simulink model "CM745A_Sci30CfgAndUse"  (R2013b)
settings: Solver=ode45  StartTime=0.0  StopTime=10.0  RelTol=1e-3
libraries: simulink x12
(part 3 of 3)

== system CM745A_Sci30CfgAndUse/Sci30CfgAndUse/Sci30CfgAndUsePer2/Sci30Transmit/If Action Subsystem1/While Iterator Subsystem/CopyRight2 ==

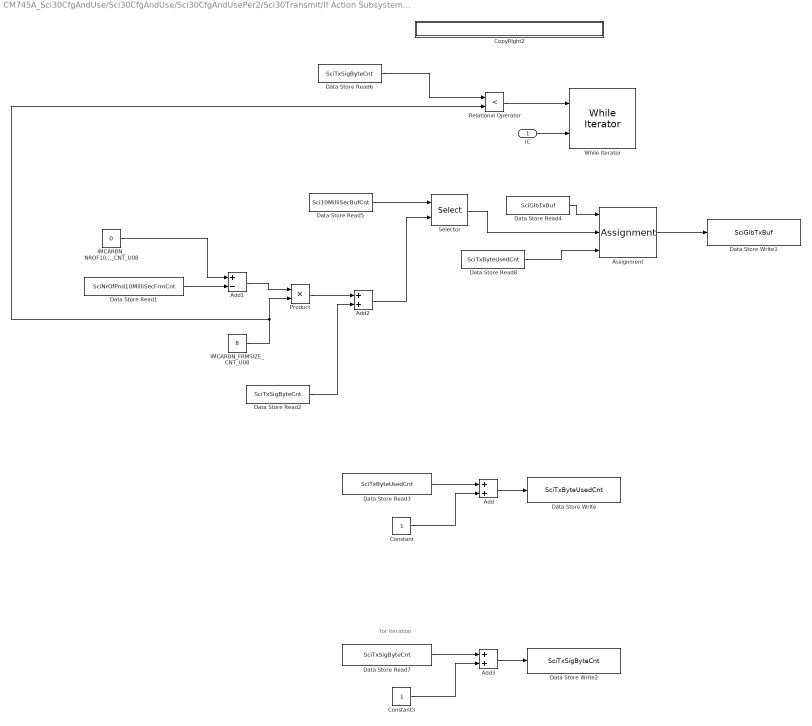
== system CM745A_Sci30CfgAndUse/Sci30CfgAndUse/Sci30CfgAndUsePer2/Sci30Transmit/If Action Subsystem1/While Iterator Subsystem/While Iterator Subsystem ==
  note: for iteration
  IC : Inport
  Add : Sum
  Add1 : Sum  Inputs=+-
  Add2 : Sum
  Add3 : Sum
  Assignment : Assignment  IndexMode=Zero-based  IndexOptions=Index vector (port)  Indices=1  OutputSizes=1
  Constant : Constant  OutDataTypeStr=uint8
  Constant3 : Constant  OutDataTypeStr=uint8
  CopyRight2 : Subsystem  Description=|  mask(Copyright Information){none=on}
      | Copyright info block.                                               
      |                                                                     
      | Place copyright information at the top of every subsystem in design.
      mask prompts: none "No parameters"
      mask help: Place copyright information at the top of every subsystem in design.
      mask Display:
      | NxtrConf = 'Nexteer Confidential';
      | 
      | sys = bdroot; %handle for the current model ("system")
      | first = get_param(sys,'Created');
      | first = first(end-3:end);  %year is last four digits
      | 
      | last = get_param(sys,'LastModifiedDate');
      | if isempty(last)
      |     last = datestr(now,'yyyy');
      | else
      |     last = last(end-3:end);
      | end
      | 
      | if strcmp(first,last)
      |     fprintf('%s -- Copyright %s Nexteer',NxtrConf,first)
      | else
      |     fprintf('%s -- %s%s- %s Nexteer',NxtrConf,char(169),first,last)
      | end
  Data Store Read1 : DataStoreRead  DataStoreName=SciNrOfPnd10MilliSecFrmCnt
  Data Store Read2 : DataStoreRead  DataStoreName=SciTxSigByteCnt
  Data Store Read3 : DataStoreRead  DataStoreName=SciTxByteUsedCnt
  Data Store Read4 : DataStoreRead  DataStoreName=SciGlbTxBuf
  Data Store Read5 : DataStoreRead  DataStoreName=Sci10MilliSecBufCnt
  Data Store Read6 : DataStoreRead  DataStoreName=SciTxSigByteCnt
  Data Store Read7 : DataStoreRead  DataStoreName=SciTxSigByteCnt
  Data Store Read8 : DataStoreRead  DataStoreName=SciTxByteUsedCnt
  Data Store Write : DataStoreWrite  DataStoreName=SciTxByteUsedCnt
  Data Store Write1 : DataStoreWrite  DataStoreName=SciGlbTxBuf
  Data Store Write2 : DataStoreWrite  DataStoreName=SciTxSigByteCnt
  IMCARBN_FRMSIZE_CNT_U08 : Constant  Value=8  OutDataTypeStr=uint8
  IMCARBN_NROF10MILLISECRATEGROUP_CNT_U08 : Constant  Value=0
  Product : Product
  Relational Operator : RelationalOperator  Operator=<  OutDataTypeStr=boolean
  Selector : Selector  IndexMode=Zero-based  InputPortWidth=2047  IndexOptions=Index vector (port)  Indices=[1 3]  OutputSizes=1
  While Iterator : WhileIterator  MaxIters=-1  ResetStates=reset
  wires:
  Data Store Read3/1 -> Add/1
  Add/1 -> Data Store Write/1
  Constant/1 -> Add/2
  Assignment/1 -> Data Store Write1/1
  Data Store Read4/1 -> Assignment/1
  Selector/1 -> Assignment/2
  Data Store Read5/1 -> Selector/1
  Add2/1 -> Selector/2
  IMCARBN_NROF10MILLISECRATEGROUP_CNT_U08/1 -> Add1/1
  Data Store Read1/1 -> Add1/2
  Add1/1 -> Product/1
  IMCARBN_FRMSIZE_CNT_U08/1 -> Relational Operator/2, Product/2
  Product/1 -> Add2/1
  Data Store Read2/1 -> Add2/2
  IC/1 -> While Iterator/2
  Data Store Read6/1 -> Relational Operator/1
  Relational Operator/1 -> While Iterator/1
  Data Store Read7/1 -> Add3/1
  Add3/1 -> Data Store Write2/1
  Constant3/1 -> Add3/2
  Data Store Read8/1 -> Assignment/3

== system CM745A_Sci30CfgAndUse/Sci30CfgAndUse/Sci30CfgAndUsePer2/Sci30Transmit/If Action Subsystem2/If Action Subsystem/CopyRight2 ==

== system CM745A_Sci30CfgAndUse/Sci30CfgAndUse/Sci30CfgAndUsePer2/Sci30Transmit/If Action Subsystem2/While Iterator Subsystem/CopyRight2 ==

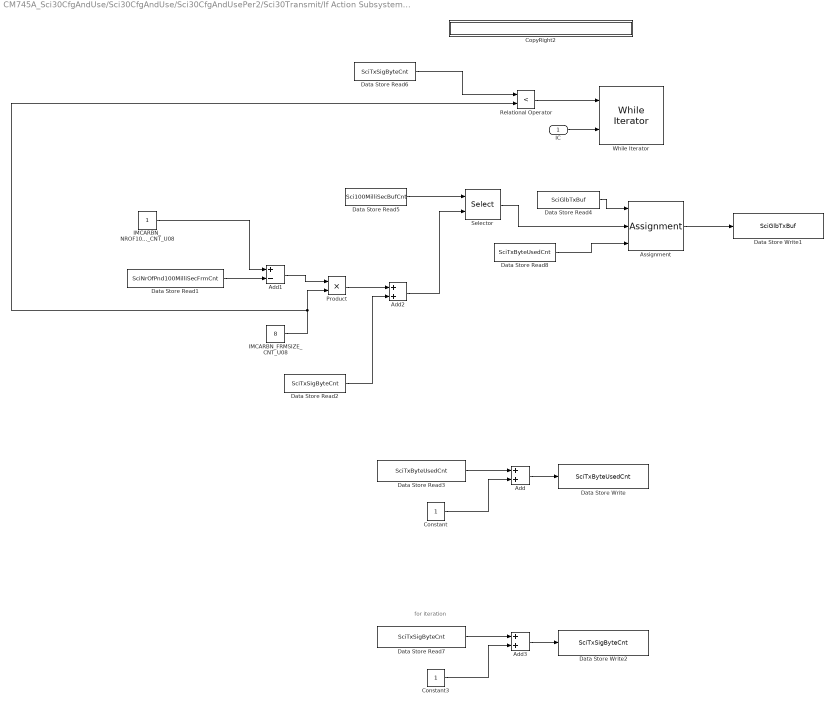
== system CM745A_Sci30CfgAndUse/Sci30CfgAndUse/Sci30CfgAndUsePer2/Sci30Transmit/If Action Subsystem2/While Iterator Subsystem/While Iterator Subsystem ==
  note: for iteration
  IC : Inport
  Add : Sum
  Add1 : Sum  Inputs=+-
  Add2 : Sum
  Add3 : Sum
  Assignment : Assignment  IndexMode=Zero-based  IndexOptions=Index vector (port)  Indices=1  OutputSizes=1
  Constant : Constant  OutDataTypeStr=uint8
  Constant3 : Constant  OutDataTypeStr=uint8
  CopyRight2 : Subsystem  Description=|  mask(Copyright Information){none=on}
      | Copyright info block.                                               
      |                                                                     
      | Place copyright information at the top of every subsystem in design.
      mask prompts: none "No parameters"
      mask help: Place copyright information at the top of every subsystem in design.
      mask Display:
      | NxtrConf = 'Nexteer Confidential';
      | 
      | sys = bdroot; %handle for the current model ("system")
      | first = get_param(sys,'Created');
      | first = first(end-3:end);  %year is last four digits
      | 
      | last = get_param(sys,'LastModifiedDate');
      | if isempty(last)
      |     last = datestr(now,'yyyy');
      | else
      |     last = last(end-3:end);
      | end
      | 
      | if strcmp(first,last)
      |     fprintf('%s -- Copyright %s Nexteer',NxtrConf,first)
      | else
      |     fprintf('%s -- %s%s- %s Nexteer',NxtrConf,char(169),first,last)
      | end
  Data Store Read1 : DataStoreRead  DataStoreName=SciNrOfPnd100MilliSecFrmCnt
  Data Store Read2 : DataStoreRead  DataStoreName=SciTxSigByteCnt
  Data Store Read3 : DataStoreRead  DataStoreName=SciTxByteUsedCnt
  Data Store Read4 : DataStoreRead  DataStoreName=SciGlbTxBuf
  Data Store Read5 : DataStoreRead  DataStoreName=Sci100MilliSecBufCnt
  Data Store Read6 : DataStoreRead  DataStoreName=SciTxSigByteCnt
  Data Store Read7 : DataStoreRead  DataStoreName=SciTxSigByteCnt
  Data Store Read8 : DataStoreRead  DataStoreName=SciTxByteUsedCnt
  Data Store Write : DataStoreWrite  DataStoreName=SciTxByteUsedCnt
  Data Store Write1 : DataStoreWrite  DataStoreName=SciGlbTxBuf
  Data Store Write2 : DataStoreWrite  DataStoreName=SciTxSigByteCnt
  IMCARBN_FRMSIZE_CNT_U08 : Constant  Value=8  OutDataTypeStr=uint8
  IMCARBN_NROF100MILLISECRATEGROUP_CNT_U08 : Constant
  Product : Product
  Relational Operator : RelationalOperator  Operator=<  OutDataTypeStr=boolean
  Selector : Selector  IndexMode=Zero-based  InputPortWidth=2047  IndexOptions=Index vector (port)  Indices=[1 3]  OutputSizes=1
  While Iterator : WhileIterator  MaxIters=-1  ResetStates=reset
  wires:
  Data Store Read3/1 -> Add/1
  Add/1 -> Data Store Write/1
  Constant/1 -> Add/2
  Assignment/1 -> Data Store Write1/1
  Data Store Read4/1 -> Assignment/1
  Selector/1 -> Assignment/2
  Data Store Read5/1 -> Selector/1
  Add2/1 -> Selector/2
  IMCARBN_NROF100MILLISECRATEGROUP_CNT_U08/1 -> Add1/1
  Data Store Read1/1 -> Add1/2
  Add1/1 -> Product/1
  IMCARBN_FRMSIZE_CNT_U08/1 -> Relational Operator/2, Product/2
  Product/1 -> Add2/1
  Data Store Read2/1 -> Add2/2
  IC/1 -> While Iterator/2
  Data Store Read6/1 -> Relational Operator/1
  Relational Operator/1 -> While Iterator/1
  Data Store Read7/1 -> Add3/1
  Add3/1 -> Data Store Write2/1
  Constant3/1 -> Add3/2
  Data Store Read8/1 -> Assignment/3

== system CM745A_Sci30CfgAndUse/Sci30CfgAndUse/Sci30CfgAndUsePer2/Sci30Transmit/Update DTS registers/If Action Subsystem/CopyRight2 ==

== system CM745A_Sci30CfgAndUse/Sci30CfgAndUse/Sci30CfgAndUsePer1/If Action Subsystem2/While Iterator Subsystem/If Action Subsystem/If Action Subsystem/CopyRight2 ==

== system CM745A_Sci30CfgAndUse/Sci30CfgAndUse/Sci30CfgAndUsePer1/If Action Subsystem2/While Iterator Subsystem/If Action Subsystem/If Action Subsystem1/CopyRight2 ==

== system CM745A_Sci30CfgAndUse/Sci30CfgAndUse/Sci30CfgAndUsePer1/If Action Subsystem2/While Iterator Subsystem/If Action Subsystem/If Action Subsystem1/RollovrAdd ==
  In1 : Inport
  In2 : Inport  Port=2
  Add : Sum
  Constant : Constant  Value=2  OutDataTypeStr=uint8
  CopyRight2 : Subsystem  Description=|  mask(Copyright Information){none=on}
      | Copyright info block.                                               
      |                                                                     
      | Place copyright information at the top of every subsystem in design.
      mask prompts: none "No parameters"
      mask help: Place copyright information at the top of every subsystem in design.
      mask Display:
      | NxtrConf = 'Nexteer Confidential';
      | 
      | sys = bdroot; %handle for the current model ("system")
      | first = get_param(sys,'Created');
      | first = first(end-3:end);  %year is last four digits
      | 
      | last = get_param(sys,'LastModifiedDate');
      | if isempty(last)
      |     last = datestr(now,'yyyy');
      | else
      |     last = last(end-3:end);
      | end
      | 
      | if strcmp(first,last)
      |     fprintf('%s -- Copyright %s Nexteer',NxtrConf,first)
      | else
      |     fprintf('%s -- %s%s- %s Nexteer',NxtrConf,char(169),first,last)
      | end
  IMCARBN_FRMSIZE_CNT_U08 : Constant  Value=8  OutDataTypeStr=uint8
  MAXSIGGROUPFORTX_CNT_U08 : Constant  Value=9  OutDataTypeStr=uint8
  Math Function : Math  Operator=mod  SaturateOnIntegerOverflow=on
  Product : Product
  Product1 : Product  OutDataTypeStr=uint8
  Out1 : Outport
  wires:
  Math Function/1 -> Out1/1
  In1/1 -> Add/1
  In2/1 -> Add/2
  Add/1 -> Math Function/1
  Constant/1 -> Product/1
  IMCARBN_FRMSIZE_CNT_U08/1 -> Product/2
  Product/1 -> Product1/1
  Product1/1 -> Math Function/2
  MAXSIGGROUPFORTX_CNT_U08/1 -> Product1/2

== system CM745A_Sci30CfgAndUse/Sci30CfgAndUse/Sci30CfgAndUsePer1/If Action Subsystem2/While Iterator Subsystem/If Action Subsystem/If Action Subsystem2/CopyRight2 ==

== system CM745A_Sci30CfgAndUse/Sci30CfgAndUse/Sci30CfgAndUsePer1/If Action Subsystem2/While Iterator Subsystem/If Action Subsystem/If Action Subsystem2/RollovrAdd ==
  In1 : Inport
  In2 : Inport  Port=2
  Add : Sum
  Constant : Constant  Value=2  OutDataTypeStr=uint8
  CopyRight2 : Subsystem  Description=|  mask(Copyright Information){none=on}
      | Copyright info block.                                               
      |                                                                     
      | Place copyright information at the top of every subsystem in design.
      mask prompts: none "No parameters"
      mask help: Place copyright information at the top of every subsystem in design.
      mask Display:
      | NxtrConf = 'Nexteer Confidential';
      | 
      | sys = bdroot; %handle for the current model ("system")
      | first = get_param(sys,'Created');
      | first = first(end-3:end);  %year is last four digits
      | 
      | last = get_param(sys,'LastModifiedDate');
      | if isempty(last)
      |     last = datestr(now,'yyyy');
      | else
      |     last = last(end-3:end);
      | end
      | 
      | if strcmp(first,last)
      |     fprintf('%s -- Copyright %s Nexteer',NxtrConf,first)
      | else
      |     fprintf('%s -- %s%s- %s Nexteer',NxtrConf,char(169),first,last)
      | end
  IMCARBN_FRMSIZE_CNT_U08 : Constant  Value=8
  MAXSIGGROUPFORTX_CNT_U08 : Constant  Value=9
  Math Function : Math  Operator=mod  SaturateOnIntegerOverflow=on
  Product : Product  OutDataTypeStr=uint8
  Product1 : Product  OutDataTypeStr=uint8
  Out1 : Outport
  wires:
  Math Function/1 -> Out1/1
  In1/1 -> Add/1
  In2/1 -> Add/2
  Add/1 -> Math Function/1
  Constant/1 -> Product/1
  IMCARBN_FRMSIZE_CNT_U08/1 -> Product/2
  Product/1 -> Product1/1
  Product1/1 -> Math Function/2
  MAXSIGGROUPFORTX_CNT_U08/1 -> Product1/2

== system CM745A_Sci30CfgAndUse/Sci30CfgAndUse/Sci30CfgAndUsePer1/If Action Subsystem2/While Iterator Subsystem/If Action Subsystem/If Action Subsystem2/RollovrAdd1 ==
  In1 : Inport
  In2 : Inport  Port=2
  Add : Sum
  Constant : Constant  Value=2  OutDataTypeStr=uint8
  CopyRight2 : Subsystem  Description=|  mask(Copyright Information){none=on}
      | Copyright info block.                                               
      |                                                                     
      | Place copyright information at the top of every subsystem in design.
      mask prompts: none "No parameters"
      mask help: Place copyright information at the top of every subsystem in design.
      mask Display:
      | NxtrConf = 'Nexteer Confidential';
      | 
      | sys = bdroot; %handle for the current model ("system")
      | first = get_param(sys,'Created');
      | first = first(end-3:end);  %year is last four digits
      | 
      | last = get_param(sys,'LastModifiedDate');
      | if isempty(last)
      |     last = datestr(now,'yyyy');
      | else
      |     last = last(end-3:end);
      | end
      | 
      | if strcmp(first,last)
      |     fprintf('%s -- Copyright %s Nexteer',NxtrConf,first)
      | else
      |     fprintf('%s -- %s%s- %s Nexteer',NxtrConf,char(169),first,last)
      | end
  IMCARBN_FRMSIZE_CNT_U08 : Constant  Value=8
  MAXSIGGROUPFORTX_CNT_U08 : Constant  Value=9
  Math Function : Math  Operator=mod  SaturateOnIntegerOverflow=on
  Product : Product
  Product1 : Product
  Out1 : Outport
  wires:
  Math Function/1 -> Out1/1
  In1/1 -> Add/1
  In2/1 -> Add/2
  Add/1 -> Math Function/1
  Constant/1 -> Product/1
  IMCARBN_FRMSIZE_CNT_U08/1 -> Product/2
  Product/1 -> Product1/1
  Product1/1 -> Math Function/2
  MAXSIGGROUPFORTX_CNT_U08/1 -> Product1/2

== system CM745A_Sci30CfgAndUse/Sci30CfgAndUse/Sci30CfgAndUsePer1/If Action Subsystem2/While Iterator Subsystem/If Action Subsystem/If Action Subsystem2/RollovrAdd2 ==
  In1 : Inport
  In2 : Inport  Port=2
  Add : Sum
  Constant : Constant  Value=2  OutDataTypeStr=uint8
  CopyRight2 : Subsystem  Description=|  mask(Copyright Information){none=on}
      | Copyright info block.                                               
      |                                                                     
      | Place copyright information at the top of every subsystem in design.
      mask prompts: none "No parameters"
      mask help: Place copyright information at the top of every subsystem in design.
      mask Display:
      | NxtrConf = 'Nexteer Confidential';
      | 
      | sys = bdroot; %handle for the current model ("system")
      | first = get_param(sys,'Created');
      | first = first(end-3:end);  %year is last four digits
      | 
      | last = get_param(sys,'LastModifiedDate');
      | if isempty(last)
      |     last = datestr(now,'yyyy');
      | else
      |     last = last(end-3:end);
      | end
      | 
      | if strcmp(first,last)
      |     fprintf('%s -- Copyright %s Nexteer',NxtrConf,first)
      | else
      |     fprintf('%s -- %s%s- %s Nexteer',NxtrConf,char(169),first,last)
      | end
  IMCARBN_FRMSIZE_CNT_U08 : Constant  Value=8
  MAXSIGGROUPFORTX_CNT_U08 : Constant  Value=9
  Math Function : Math  Operator=mod  SaturateOnIntegerOverflow=on
  Product : Product
  Product1 : Product
  Out1 : Outport
  wires:
  MAXSIGGROUPFORTX_CNT_U08/1 -> Product1/2
  Product1/1 -> Math Function/2
  Product/1 -> Product1/1
  IMCARBN_FRMSIZE_CNT_U08/1 -> Product/2
  Constant/1 -> Product/1
  Add/1 -> Math Function/1
  In2/1 -> Add/2
  In1/1 -> Add/1
  Math Function/1 -> Out1/1

== system CM745A_Sci30CfgAndUse/Sci30CfgAndUse/Sci30CfgAndUsePer1/If Action Subsystem2/While Iterator Subsystem/If Action Subsystem/If Action Subsystem2/RollovrAdd3 ==
  In1 : Inport
  In2 : Inport  Port=2
  Add : Sum
  Constant : Constant  Value=2  OutDataTypeStr=uint8
  CopyRight2 : Subsystem  Description=|  mask(Copyright Information){none=on}
      | Copyright info block.                                               
      |                                                                     
      | Place copyright information at the top of every subsystem in design.
      mask prompts: none "No parameters"
      mask help: Place copyright information at the top of every subsystem in design.
      mask Display:
      | NxtrConf = 'Nexteer Confidential';
      | 
      | sys = bdroot; %handle for the current model ("system")
      | first = get_param(sys,'Created');
      | first = first(end-3:end);  %year is last four digits
      | 
      | last = get_param(sys,'LastModifiedDate');
      | if isempty(last)
      |     last = datestr(now,'yyyy');
      | else
      |     last = last(end-3:end);
      | end
      | 
      | if strcmp(first,last)
      |     fprintf('%s -- Copyright %s Nexteer',NxtrConf,first)
      | else
      |     fprintf('%s -- %s%s- %s Nexteer',NxtrConf,char(169),first,last)
      | end
  IMCARBN_FRMSIZE_CNT_U08 : Constant  Value=8
  MAXSIGGROUPFORTX_CNT_U08 : Constant  Value=9
  Math Function : Math  Operator=mod  SaturateOnIntegerOverflow=on
  Product : Product
  Product1 : Product
  Out1 : Outport
  wires:
  Math Function/1 -> Out1/1
  In1/1 -> Add/1
  In2/1 -> Add/2
  Add/1 -> Math Function/1
  Constant/1 -> Product/1
  IMCARBN_FRMSIZE_CNT_U08/1 -> Product/2
  Product/1 -> Product1/1
  Product1/1 -> Math Function/2
  MAXSIGGROUPFORTX_CNT_U08/1 -> Product1/2

== system CM745A_Sci30CfgAndUse/Sci30CfgAndUse/Sci30CfgAndUsePer1/If Action Subsystem2/While Iterator Subsystem/If Action Subsystem/If Action Subsystem2/RollovrAdd4 ==
  In1 : Inport
  In2 : Inport  Port=2
  Add : Sum
  Constant : Constant  Value=2  OutDataTypeStr=uint8
  CopyRight2 : Subsystem  Description=|  mask(Copyright Information){none=on}
      | Copyright info block.                                               
      |                                                                     
      | Place copyright information at the top of every subsystem in design.
      mask prompts: none "No parameters"
      mask help: Place copyright information at the top of every subsystem in design.
      mask Display:
      | NxtrConf = 'Nexteer Confidential';
      | 
      | sys = bdroot; %handle for the current model ("system")
      | first = get_param(sys,'Created');
      | first = first(end-3:end);  %year is last four digits
      | 
      | last = get_param(sys,'LastModifiedDate');
      | if isempty(last)
      |     last = datestr(now,'yyyy');
      | else
      |     last = last(end-3:end);
      | end
      | 
      | if strcmp(first,last)
      |     fprintf('%s -- Copyright %s Nexteer',NxtrConf,first)
      | else
      |     fprintf('%s -- %s%s- %s Nexteer',NxtrConf,char(169),first,last)
      | end
  IMCARBN_FRMSIZE_CNT_U08 : Constant  Value=8
  MAXSIGGROUPFORTX_CNT_U08 : Constant  Value=9
  Math Function : Math  Operator=mod  SaturateOnIntegerOverflow=on
  Product : Product
  Product1 : Product
  Out1 : Outport
  wires:
  MAXSIGGROUPFORTX_CNT_U08/1 -> Product1/2
  Product1/1 -> Math Function/2
  Product/1 -> Product1/1
  IMCARBN_FRMSIZE_CNT_U08/1 -> Product/2
  Constant/1 -> Product/1
  Add/1 -> Math Function/1
  In2/1 -> Add/2
  In1/1 -> Add/1
  Math Function/1 -> Out1/1

== system CM745A_Sci30CfgAndUse/Sci30CfgAndUse/Sci30CfgAndUsePer1/If Action Subsystem2/While Iterator Subsystem/If Action Subsystem/If Action Subsystem2/RollovrAdd5 ==
  In1 : Inport
  In2 : Inport  Port=2
  Add : Sum
  Constant : Constant  Value=2  OutDataTypeStr=uint8
  CopyRight2 : Subsystem  Description=|  mask(Copyright Information){none=on}
      | Copyright info block.                                               
      |                                                                     
      | Place copyright information at the top of every subsystem in design.
      mask prompts: none "No parameters"
      mask help: Place copyright information at the top of every subsystem in design.
      mask Display:
      | NxtrConf = 'Nexteer Confidential';
      | 
      | sys = bdroot; %handle for the current model ("system")
      | first = get_param(sys,'Created');
      | first = first(end-3:end);  %year is last four digits
      | 
      | last = get_param(sys,'LastModifiedDate');
      | if isempty(last)
      |     last = datestr(now,'yyyy');
      | else
      |     last = last(end-3:end);
      | end
      | 
      | if strcmp(first,last)
      |     fprintf('%s -- Copyright %s Nexteer',NxtrConf,first)
      | else
      |     fprintf('%s -- %s%s- %s Nexteer',NxtrConf,char(169),first,last)
      | end
  IMCARBN_FRMSIZE_CNT_U08 : Constant  Value=8
  MAXSIGGROUPFORTX_CNT_U08 : Constant  Value=9
  Math Function : Math  Operator=mod  SaturateOnIntegerOverflow=on
  Product : Product
  Product1 : Product
  Out1 : Outport
  wires:
  Math Function/1 -> Out1/1
  In1/1 -> Add/1
  In2/1 -> Add/2
  Add/1 -> Math Function/1
  Constant/1 -> Product/1
  IMCARBN_FRMSIZE_CNT_U08/1 -> Product/2
  Product/1 -> Product1/1
  Product1/1 -> Math Function/2
  MAXSIGGROUPFORTX_CNT_U08/1 -> Product1/2

== system CM745A_Sci30CfgAndUse/Sci30CfgAndUse/Sci30CfgAndUsePer1/If Action Subsystem2/While Iterator Subsystem/If Action Subsystem/If Action Subsystem2/RollovrAdd6 ==
  In1 : Inport
  In2 : Inport  Port=2
  Add : Sum
  Constant : Constant  Value=2  OutDataTypeStr=uint8
  CopyRight2 : Subsystem  Description=|  mask(Copyright Information){none=on}
      | Copyright info block.                                               
      |                                                                     
      | Place copyright information at the top of every subsystem in design.
      mask prompts: none "No parameters"
      mask help: Place copyright information at the top of every subsystem in design.
      mask Display:
      | NxtrConf = 'Nexteer Confidential';
      | 
      | sys = bdroot; %handle for the current model ("system")
      | first = get_param(sys,'Created');
      | first = first(end-3:end);  %year is last four digits
      | 
      | last = get_param(sys,'LastModifiedDate');
      | if isempty(last)
      |     last = datestr(now,'yyyy');
      | else
      |     last = last(end-3:end);
      | end
      | 
      | if strcmp(first,last)
      |     fprintf('%s -- Copyright %s Nexteer',NxtrConf,first)
      | else
      |     fprintf('%s -- %s%s- %s Nexteer',NxtrConf,char(169),first,last)
      | end
  IMCARBN_FRMSIZE_CNT_U08 : Constant  Value=8
  MAXSIGGROUPFORTX_CNT_U08 : Constant  Value=9
  Math Function : Math  Operator=mod  SaturateOnIntegerOverflow=on
  Product : Product
  Product1 : Product
  Out1 : Outport
  wires:
  MAXSIGGROUPFORTX_CNT_U08/1 -> Product1/2
  Product1/1 -> Math Function/2
  Product/1 -> Product1/1
  IMCARBN_FRMSIZE_CNT_U08/1 -> Product/2
  Constant/1 -> Product/1
  Add/1 -> Math Function/1
  In2/1 -> Add/2
  In1/1 -> Add/1
  Math Function/1 -> Out1/1

== system CM745A_Sci30CfgAndUse/Sci30CfgAndUse/Sci30CfgAndUsePer1/If Action Subsystem2/While Iterator Subsystem/If Action Subsystem/If Action Subsystem2/RollovrAdd7 ==
  In1 : Inport
  In2 : Inport  Port=2
  Add : Sum
  Constant : Constant  Value=2  OutDataTypeStr=uint8
  CopyRight2 : Subsystem  Description=|  mask(Copyright Information){none=on}
      | Copyright info block.                                               
      |                                                                     
      | Place copyright information at the top of every subsystem in design.
      mask prompts: none "No parameters"
      mask help: Place copyright information at the top of every subsystem in design.
      mask Display:
      | NxtrConf = 'Nexteer Confidential';
      | 
      | sys = bdroot; %handle for the current model ("system")
      | first = get_param(sys,'Created');
      | first = first(end-3:end);  %year is last four digits
      | 
      | last = get_param(sys,'LastModifiedDate');
      | if isempty(last)
      |     last = datestr(now,'yyyy');
      | else
      |     last = last(end-3:end);
      | end
      | 
      | if strcmp(first,last)
      |     fprintf('%s -- Copyright %s Nexteer',NxtrConf,first)
      | else
      |     fprintf('%s -- %s%s- %s Nexteer',NxtrConf,char(169),first,last)
      | end
  IMCARBN_FRMSIZE_CNT_U08 : Constant  Value=8
  MAXSIGGROUPFORTX_CNT_U08 : Constant  Value=9
  Math Function : Math  Operator=mod  SaturateOnIntegerOverflow=on
  Product : Product
  Product1 : Product
  Out1 : Outport
  wires:
  Math Function/1 -> Out1/1
  In1/1 -> Add/1
  In2/1 -> Add/2
  Add/1 -> Math Function/1
  Constant/1 -> Product/1
  IMCARBN_FRMSIZE_CNT_U08/1 -> Product/2
  Product/1 -> Product1/1
  Product1/1 -> Math Function/2
  MAXSIGGROUPFORTX_CNT_U08/1 -> Product1/2

== system CM745A_Sci30CfgAndUse/Sci30CfgAndUse/Sci30CfgAndUsePer1/If Action Subsystem2/While Iterator Subsystem/If Action Subsystem/If Action Subsystem2/RollovrAdd8 ==
  In1 : Inport
  In2 : Inport  Port=2
  Add : Sum
  Constant : Constant  Value=2  OutDataTypeStr=uint8
  CopyRight2 : Subsystem  Description=|  mask(Copyright Information){none=on}
      | Copyright info block.                                               
      |                                                                     
      | Place copyright information at the top of every subsystem in design.
      mask prompts: none "No parameters"
      mask help: Place copyright information at the top of every subsystem in design.
      mask Display:
      | NxtrConf = 'Nexteer Confidential';
      | 
      | sys = bdroot; %handle for the current model ("system")
      | first = get_param(sys,'Created');
      | first = first(end-3:end);  %year is last four digits
      | 
      | last = get_param(sys,'LastModifiedDate');
      | if isempty(last)
      |     last = datestr(now,'yyyy');
      | else
      |     last = last(end-3:end);
      | end
      | 
      | if strcmp(first,last)
      |     fprintf('%s -- Copyright %s Nexteer',NxtrConf,first)
      | else
      |     fprintf('%s -- %s%s- %s Nexteer',NxtrConf,char(169),first,last)
      | end
  IMCARBN_FRMSIZE_CNT_U08 : Constant  Value=8
  MAXSIGGROUPFORTX_CNT_U08 : Constant  Value=9
  Math Function : Math  Operator=mod  SaturateOnIntegerOverflow=on
  Product : Product
  Product1 : Product
  Out1 : Outport
  wires:
  MAXSIGGROUPFORTX_CNT_U08/1 -> Product1/2
  Product1/1 -> Math Function/2
  Product/1 -> Product1/1
  IMCARBN_FRMSIZE_CNT_U08/1 -> Product/2
  Constant/1 -> Product/1
  Add/1 -> Math Function/1
  In2/1 -> Add/2
  In1/1 -> Add/1
  Math Function/1 -> Out1/1

== system CM745A_Sci30CfgAndUse/Sci30CfgAndUse/Sci30CfgAndUsePer1/If Action Subsystem2/While Iterator Subsystem/If Action Subsystem/If Action Subsystem2/SetRxSigGroup ==
  In1 : Inport
  In2 : Inport  Port=2
  CopyRight2 : Subsystem  Description=|  mask(Copyright Information){none=on}
      | Copyright info block.                                               
      |                                                                     
      | Place copyright information at the top of every subsystem in design.
      mask prompts: none "No parameters"
      mask help: Place copyright information at the top of every subsystem in design.
      mask Display:
      | NxtrConf = 'Nexteer Confidential';
      | 
      | sys = bdroot; %handle for the current model ("system")
      | first = get_param(sys,'Created');
      | first = first(end-3:end);  %year is last four digits
      | 
      | last = get_param(sys,'LastModifiedDate');
      | if isempty(last)
      |     last = datestr(now,'yyyy');
      | else
      |     last = last(end-3:end);
      | end
      | 
      | if strcmp(first,last)
      |     fprintf('%s -- Copyright %s Nexteer',NxtrConf,first)
      | else
      |     fprintf('%s -- %s%s- %s Nexteer',NxtrConf,char(169),first,last)
      | end
  Terminator : Terminator
  Terminator1 : Terminator
  wires:
  In2/1 -> Terminator1/1
  In1/1 -> Terminator/1

== system CM745A_Sci30CfgAndUse/Sci30CfgAndUse/Sci30CfgAndUsePer1/If Action Subsystem2/While Iterator Subsystem/If Action Subsystem/RollovrAdd/CopyRight2 ==

== system CM745A_Sci30CfgAndUse/Sci30CfgAndUse/Sci30CfgAndUsePer1/If Action Subsystem2/While Iterator Subsystem/If Action Subsystem1/RollovrAdd/CopyRight2 ==

== system CM745A_Sci30CfgAndUse/Sci30CfgAndUse/Sci30CfgAndUsePer2/Sci30Transmit/If Action Subsystem1/While Iterator Subsystem/While Iterator Subsystem/CopyRight2 ==

== system CM745A_Sci30CfgAndUse/Sci30CfgAndUse/Sci30CfgAndUsePer2/Sci30Transmit/If Action Subsystem2/While Iterator Subsystem/While Iterator Subsystem/CopyRight2 ==

== system CM745A_Sci30CfgAndUse/Sci30CfgAndUse/Sci30CfgAndUsePer1/If Action Subsystem2/While Iterator Subsystem/If Action Subsystem/If Action Subsystem1/RollovrAdd/CopyRight2 ==

== system CM745A_Sci30CfgAndUse/Sci30CfgAndUse/Sci30CfgAndUsePer1/If Action Subsystem2/While Iterator Subsystem/If Action Subsystem/If Action Subsystem2/RollovrAdd/CopyRight2 ==

== system CM745A_Sci30CfgAndUse/Sci30CfgAndUse/Sci30CfgAndUsePer1/If Action Subsystem2/While Iterator Subsystem/If Action Subsystem/If Action Subsystem2/RollovrAdd1/CopyRight2 ==

== system CM745A_Sci30CfgAndUse/Sci30CfgAndUse/Sci30CfgAndUsePer1/If Action Subsystem2/While Iterator Subsystem/If Action Subsystem/If Action Subsystem2/RollovrAdd2/CopyRight2 ==

== system CM745A_Sci30CfgAndUse/Sci30CfgAndUse/Sci30CfgAndUsePer1/If Action Subsystem2/While Iterator Subsystem/If Action Subsystem/If Action Subsystem2/RollovrAdd3/CopyRight2 ==

== system CM745A_Sci30CfgAndUse/Sci30CfgAndUse/Sci30CfgAndUsePer1/If Action Subsystem2/While Iterator Subsystem/If Action Subsystem/If Action Subsystem2/RollovrAdd4/CopyRight2 ==

== system CM745A_Sci30CfgAndUse/Sci30CfgAndUse/Sci30CfgAndUsePer1/If Action Subsystem2/While Iterator Subsystem/If Action Subsystem/If Action Subsystem2/RollovrAdd5/CopyRight2 ==

== system CM745A_Sci30CfgAndUse/Sci30CfgAndUse/Sci30CfgAndUsePer1/If Action Subsystem2/While Iterator Subsystem/If Action Subsystem/If Action Subsystem2/RollovrAdd6/CopyRight2 ==

== system CM745A_Sci30CfgAndUse/Sci30CfgAndUse/Sci30CfgAndUsePer1/If Action Subsystem2/While Iterator Subsystem/If Action Subsystem/If Action Subsystem2/RollovrAdd7/CopyRight2 ==

== system CM745A_Sci30CfgAndUse/Sci30CfgAndUse/Sci30CfgAndUsePer1/If Action Subsystem2/While Iterator Subsystem/If Action Subsystem/If Action Subsystem2/RollovrAdd8/CopyRight2 ==

== system CM745A_Sci30CfgAndUse/Sci30CfgAndUse/Sci30CfgAndUsePer1/If Action Subsystem2/While Iterator Subsystem/If Action Subsystem/If Action Subsystem2/SetRxSigGroup/CopyRight2 ==
